simulink model "first_order_second_order_open_close_loop_simulink"  (R2022b)
settings: Solver=VariableStepAuto  StartTime=0.0  StopTime=10.0  RelTol=1e-3
settings Model: Creator=yasso  LastModifiedBy=yasso

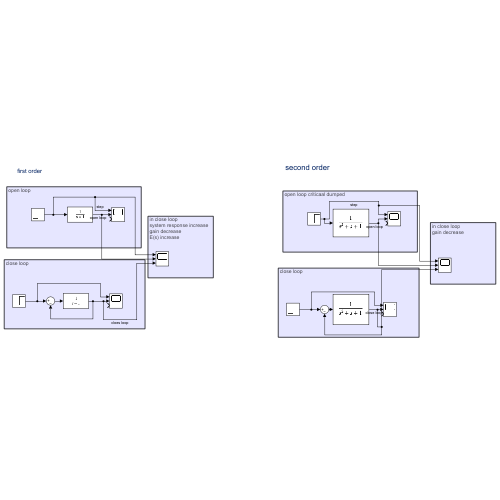
[thumbnail: Simulink's stored preview of the top-level diagram]
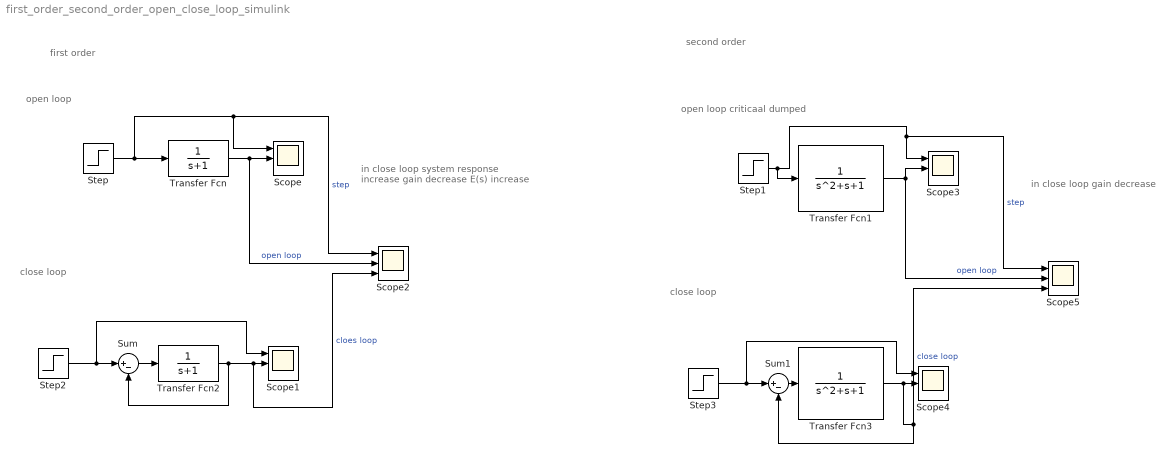
== system first_order_second_order_open_close_loop_simulink ==
  note: first order
  note: in close loop
      | system response increase
      | gain decrease
      | E(s) increase
  note: close loop
  note: open loop
  note: open loop criticaal dumped
  note: close loop
  note: in close loop
      | gain decrease
  note: second order
  Scope{,1..5} (6 alike) : Scope  NumInputPorts=3
  Step{,1..3} (4 alike) : Step  SampleTime=0
  Sum : Sum  Inputs=|+-
  Sum1 : Sum  Inputs=|+-
  Transfer Fcn : TransferFcn  Numerator=1  Denominator=[1 1]
  Transfer Fcn1 : TransferFcn  Numerator=1  Denominator=[1 1 1]
  Transfer Fcn2 : TransferFcn  Numerator=1  Denominator=[1 1]
  Transfer Fcn3 : TransferFcn  Numerator=1  Denominator=[1 1 1]
  wires:
  Transfer Fcn1/1 -> Scope3/2, Scope5/2  "open loop"
  Step1/1 -> Transfer Fcn1/1, Scope3/1, Scope5/1  "step"
  Transfer Fcn3/1 -> Scope4/2, Sum1/2, Scope5/3  "close loop"
  Step3/1 -> Scope4/1, Sum1/1
  Sum1/1 -> Transfer Fcn3/1
  Transfer Fcn2/1 -> Scope1/2, Scope2/3, Sum/2  "cloes loop"
  Step/1 -> Transfer Fcn/1, Scope2/1, Scope/1  "step"
  Sum/1 -> Transfer Fcn2/1
  Transfer Fcn/1 -> Scope/2, Scope2/2  "open loop"
  Step2/1 -> Sum/1, Scope1/1
